simulink model "EOM_example_y_fb_2015"  (R2015b)
settings: Solver=ode5  StartTime=0.0  StopTime=50  FixedStep=0.01  RelTol=1e-3
InitFcn:
  | load data
undefined symbols (not defined in the file or in its folder): k
settings Model: Creator=isaackaminer  LastModifiedBy=jaschnie
settings DataIOCC: ExternalInput=[0 1.16868359536618 0.460083528356531]  InitialState=[]  LoadExternalInput=on  LoadInitialState=on  SaveFormat=Array
settings OptimizationCC: DefaultParameterBehavior=Inlined  BufferReuse=off
settings DebuggingCC: SolverPrmCheckMsg=warning  AllowSymbolicDim=on  InitInArrayFormatMsg=none
settings HardwareCC: ProdBitPerPointer=32  ProdLargestAtomicFloat=None  ProdIntDivRoundTo=Undefined  ProdEndianess=Unspecified  ProdWordSize=32  ProdHWDeviceType=32-bit Generic
settings GRTTargetCC: GeneratePreprocessorConditionals=Disable all
settings ConfigComp: CovModelRefEnable=Off  CovSFcnEnable=off

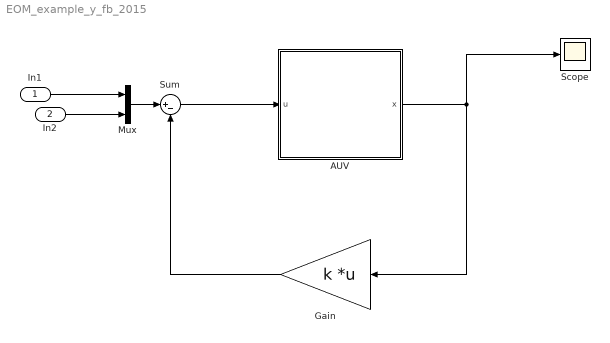
== system EOM_example_y_fb_2015 ==
  In1 : Inport
  In2 : Inport  Port=2
  AUV : Subsystem
  Gain : Gain  Gain=k  Multiplication=Matrix(K*u)
  Mux : Mux  Inputs=2
  Scope : Scope
  Sum : Sum  Inputs=|+-
  wires:
  AUV/1(x) -> Scope/1, Gain/1
  Sum/1 -> AUV/1(u)
  Gain/1 -> Sum/2
  Mux/1 -> Sum/1
  In1/1 -> Mux/1
  In2/1 -> Mux/2

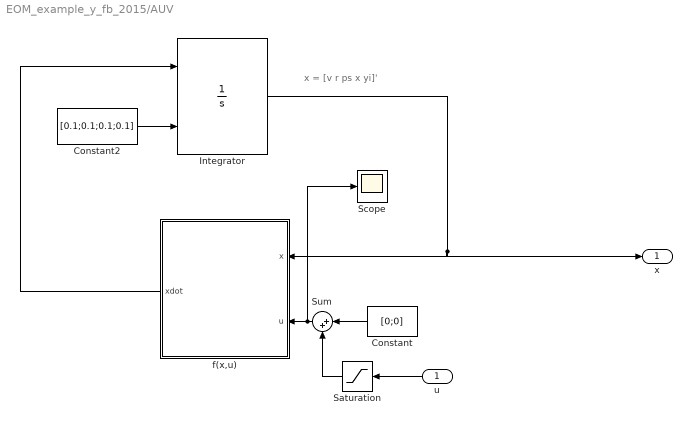
== system EOM_example_y_fb_2015/AUV ==
  note: x = [v r ps x yi]'
  u : Inport
  Constant : Constant  Value=[0;0]
  Constant2 : Constant  Value=[0.1;0.1;0.1;0.1]
  Integrator : Integrator  InitialConditionSource=external
  Saturation : Saturate  UpperLimit=5  LowerLimit=-5
  Scope : Scope
  Sum : Sum  Inputs=|++
  f(x,u) : MATLAB Function  TreatAsAtomicUnit=on
  x : Outport
  wires:
  f(x,u)/1(xdot) -> Integrator/1
  Integrator/1 -> x/1, f(x,u)/1(x)
  Constant2/1 -> Integrator/2
  Constant/1 -> Sum/1
  Sum/1 -> Scope/1, f(x,u)/2(u)
  u/1 -> Saturation/1
  Saturation/1 -> Sum/2

== matlab function EOM_example_y_fb_2015/AUV/f(x,u) ==
  data: x input; xdot output; u input
function xdot = fcn(x,u)
%#codegen

% Sub parameters
m = .0358;
Iz = .0022;
xg = .0014;
Yrdot = -.00178;
Yr = .01187;
Yv = -.107;
Yvdot = -.0343;
Ydb = .01241;
Yds = Ydb;
Nrdot = -.00047;
Nvdot = -.00178;
Nr = -.0039;
Nv = -.00769;
Nds = -.0047;
Ndb = .0035;
   
% x = [v r psi x y]
% u = [u_1 u_2]

v = x(1); r = x(2); psi = x(3); y1 = x(4);

db = u(1); ds = u(2);

M = [  (m - Yvdot)  (m*xg - Yrdot) 0 0;
     (m*xg - Nvdot)  (Iz - Nrdot)  0 0;
           0              0        1 0;
           0              0        0 1];

xdot = M \[Yv*v + Yr*r + Ydb*db + Yds*ds; % Y-force eqn
           Nv*v + Nr*r + Ndb*db + Nds*ds; % N-moment eqn
           r;
           sin(psi) + v*cos(psi)];
